simulink model "testSystemObject"  (R2024a)
settings: Solver=FixedStepAuto  StartTime=0.0  StopTime=250  RelTol=1e-3
settings Model: Creator=The MathWorks, Inc.  LastModifiedBy=csamak
settings SolverCC: AlgebraicLoopSolver=TrustRegion
settings DebuggingCC: UnconnectedInputMsg=warning  UnconnectedOutputMsg=warning  UnconnectedLineMsg=warning
settings ModelReferenceCC: EnableRefExpFcnMdlSchedulingChecks=on
settings RTWCC: GPUComputeCapability=3.5

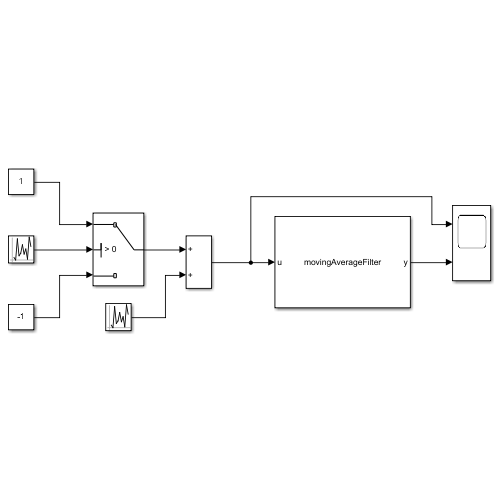
[thumbnail: Simulink's stored preview of the top-level diagram]
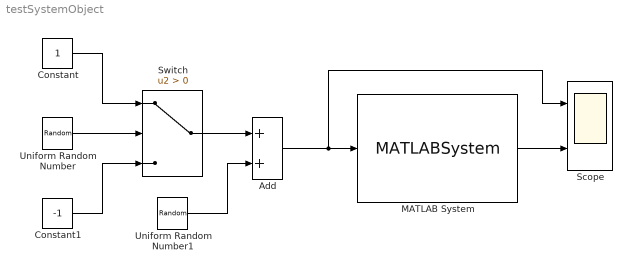
== system testSystemObject ==
  Add : Sum
  Constant : Constant  VectorParams1D=off  SampleTime=1
  Constant1 : Constant  Value=-1  SampleTime=1
  MATLAB System : MATLABSystem  System=movingAverageFilter  WindowLength=5  SimulateUsing=Code generation
      mask Type: movingAverageFilter
      mask Display:
      | disp('movingAverageFilter');
      | port_label('input',1,'u');
      | port_label('output',1,'y');
  Scope : Scope  NumInputPorts=2
  Switch : Switch  Criteria=u2 > Threshold  SaturateOnIntegerOverflow=off  InputSameDT=off
  Uniform Random Number : UniformRandomNumber  SampleTime=1  VectorParams1D=off
  Uniform Random Number1 : UniformRandomNumber  SampleTime=1  VectorParams1D=off
  wires:
  Add/1 -> MATLAB System/1, Scope/1
  MATLAB System/1 -> Scope/2
  Constant/1 -> Switch/1
  Uniform Random Number/1 -> Switch/2
  Constant1/1 -> Switch/3
  Switch/1 -> Add/1
  Uniform Random Number1/1 -> Add/2
